simulink model "drawWorks_Sim_DriveBlk"  (R2017b)
settings: Solver=ode23t  StartTime=0.0  StopTime=30  FixedStep=Ts  MaxStep=1e-4  RelTol=1e-3  AbsTol=1e-3  EnableMultiTasking=on
PreLoadFcn:
  | addpath('./Images');
  | addpath('./Simscape_Pulley_Library');
InitFcn:
  | DrawworksParameters();
values from neighbouring files (symbols this model uses):
  n = 6    [DrawworksParameters.m]
  Ts = 1.5e-4    (= 0.00015)    [DrawworksParameters.m]
  Tssc = 10*Ts    (= 0.0015)    [DrawworksParameters.m]
undefined symbols (not defined in the file or in its folder): Drum, Tackle
libraries: fl_lib x19, CustomComponents_lib x11, nesl_utility x5, sdl_lib x3, powerlib x2, electricdrivelib x1
Description:
  | Copyright 2008-2016 The MathWorks, Inc.
settings Model: ExtModeAutoUpdateStatusClock=off  Creator=MathWorks  LastModifiedBy=jlesage
settings DataIOCC: LimitDataPoints=on  SaveFormat=Array  SignalLoggingSaveFormat=ModelDataLogs  SaveOutput=off  SignalLogging=off  SaveTime=off  SignalLoggingName=sigsOut
settings OptimizationCC: ExpressionDepthLimit=2147483647  InitFltsAndDblsToZero=on  LifeSpan=inf
settings DebuggingCC: UnderspecifiedInitializationDetection=Classic  MergeDetectMultiDrivingBlocksExec=none  CheckExecutionContextPreStartOutputMsg=on  CheckExecutionContextRuntimeOutputMsg=on  SignalResolutionControl=TryResolveAllWithWarning  MultiTaskDSMMsg=warning  MultiTaskCondExecSysMsg=none  FcnCallInpInsideContextMsg=warning  StateNameClashWarn=warning  SFUnexpectedBacktrackingDiag=warning  SFNoUnconditionalDefaultTransitionDiag=warning  SFExecutionAtInitializationDiag=none
settings HardwareCC: ProdBitPerPointer=32  ProdBitPerSizeT=32  ProdBitPerPtrDiffT=32  ProdLargestAtomicFloat=None  ProdIntDivRoundTo=Undefined  ProdEndianess=Unspecified  ProdWordSize=32  ProdHWDeviceType=32-bit Generic  TargetUnknown=on
settings ModelReferenceCC: PropagateSignalLabelsOutOfModel=off
settings CodeAppCC: StateflowObjectComments=on
settings GRTTargetCC: TargetLangStandard=C89/C90 (ANSI)  GeneratePreprocessorConditionals=Disable all  CombineOutputUpdateFcns=off  GRTInterface=on
settings ConfigComp: CovMetricSettings=dw  CovHtmlReporting=on  CovSaveCumulativeToWorkspaceVar=on  CovSaveSingleToWorkspaceVar=on  CovExternalEMLEnable=off  CovSFcnEnable=off
settings SimscapeCC: SimscapeNormalizeSystem=off

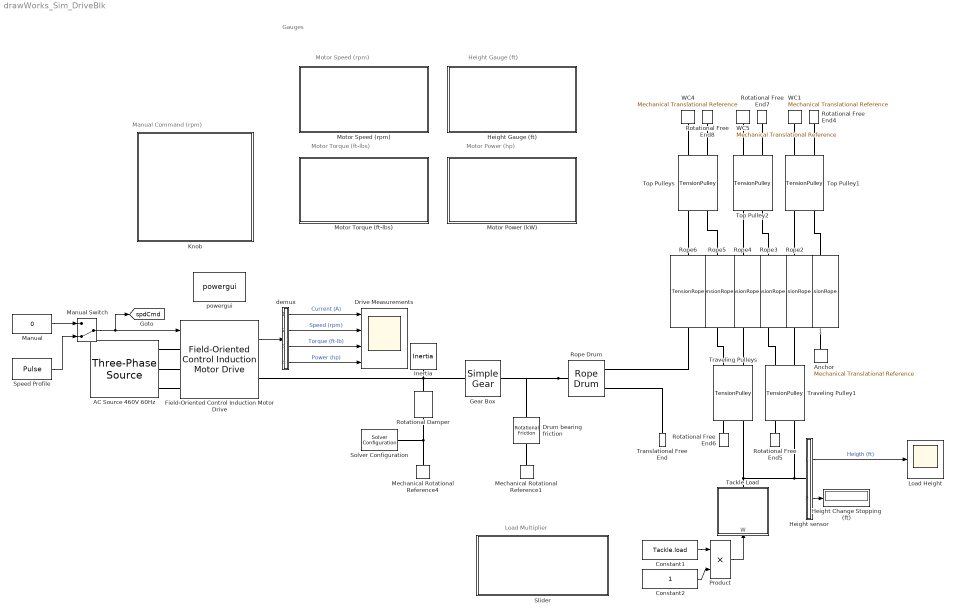
== system drawWorks_Sim_DriveBlk ==
  note: Gauges
  note: Motor Speed (rpm)
  note: Height Gauge (ft)
  note: Motor Torque (ft-lbs)
  note: Motor Power (hp)
  note: Manual Command (rpm)
  note: Load Multiplier
  1 : CustomComponents_lib/TensionRope  rope_stiff=Rope.stiffness N/m  damping=Rope.damping N/(m/s)  L0=10 m  mass=1 kg  s_specify=off  s_priority=High  s=0.08 m  s_nominal_specify=off  s_nominal_unit=m  s_nominal_value=1  L_specify=off  L_priority=High  L=1 m  L_nominal_specify=off  L_nominal_unit=m  L_nominal_value=1  f_specify=on  f_priority=High  f=Tackle.load/n N  f_nominal_specify=off  f_nominal_unit=N  f_nominal_value=1  v_specify=off  v_priority=High  v=0 m/s  v_nominal_specify=off  v_nominal_unit=m/s  v_nominal_value=1  fd_specify=off  fd_priority=High  fd=0 N  fd_nominal_specify=off  fd_nominal_unit=N  fd_nominal_value=1  fs_specify=off  fs_priority=High  fs=0 N  fs_nominal_specify=off  fs_nominal_unit=N  fs_nominal_value=1
  AC Source 460V 60Hz : powerlib/Electrical Sources/Three-Phase Source  InternalConnection=Yg  VoltagePhases=off  Voltage=2300  PhaseAngle=0  Voltage_phases=[25e3 25e3 25e3]/sqrt(3)  PhaseAngles_phases=[0 -120 +120]  Frequency=60  NonIdealSource=on  SpecifyImpedance=off  Resistance=0.02  Inductance=0.05e-3  ShortCircuitLevel=100e6  BaseVoltage=25e3  XRratio=7  BusType=swing  Pref=0  Qref=0  Prefabc=[10e3, 10e3, 10e3]  Qrefabc=[0, 0, 0]  Qmin=-inf  Qmax=inf
  Anchor : fl_lib/Mechanical/Translational Elements/Mechanical Translational Reference
  Constant1 : Constant  Value=Tackle.load
  Constant2 : Constant
  Drive Measurements : Scope  NumInputPorts=4
  Drum bearing friction : fl_lib/Mechanical/Rotational Elements/Rotational Friction  brkwy_trq=Drum.friction*1.1 N*m  brkwy_vel=0.060623 rad/s  Col_trq=Drum.friction N*m  visc_coef=Drum.viscous N*m/(rad/s)  w_specify=on  w_priority=Low  w=0 rad/s  w_nominal_specify=off  w_nominal_unit=rad/s  w_nominal_value=1  t_specify=off  t_priority=High  t=0 N*m  t_nominal_specify=off  t_nominal_unit=N*m  t_nominal_value=1
      settings: SourceProductName=Simscape
  Field-Oriented Control Induction Motor Drive : electricdrivelib/AC drives/Field-Oriented Control Induction Motor Drive  ReferenceFrame=Rotor  IterativeDiscreteModel=Forward Euler  Pn=2250*746  Vn=2300  fn=60  Rs=0.029  Lls=0.226/(2*pi*60)  Lms=13.04/(2*pi*60)  Rr=0.022  Llr=0.226/(2*pi*60)  ia=0  pha=0  ib=0  phb=0  ic=0  phc=0  J=3.1  Friction=0.08  p=2  slip=1  thdeg=0  Rsnb_rec=10e3  Csnb_rec=20e-9  Ron_rec=1e-3  Vf_rec=1.3  cap_bus=7500e-6  Rbrake=8  fbrake=4000  activationVoltage=700  shutdownVoltage=660  sourceFrequency=60  deviceType=IGBT / Diodes  Ron_inv=1e-3  Vf_inv=0.8  Vfd_inv=0.8  Tf=1e-6  Tt=2e-6  Tf_GTO=10e-6  Tt_GTO=20e-6  Rsnb_inv=5e3  Csnb_inv=inf  regulationType=Speed regulation  Acc=750  Dec=-750  kp_sc=300  ki_sc=2000  fc_sc=1000  Tsc=Ts  Tmin=-30000  Tmax=30000  in_flux=0.73  nf=0.73  kp_fc=50  ki_fc=30  freqc_fc=27  fluxmin=-2  fluxmax=2  modulationType=Hysteresis  h=10  kp_Id=5  ki_Id=100  kp_Iq=5  ki_Iq=100  fc_bus=50  car_freq=20000  freq_max=20000  Tvect=Ts  baseSampleTime=Ts  outputBusMode=Single output bus  busLabels=off  MechanicalLoad=Mechanical rotational port  modelDetailLevel=Average  driveType=AC3  AverageValue=on
      settings: SourceProductName=Simscape Power Systems  SourceProductBaseCode=PS
  Gear Box : sdl_lib/Gears/Simple Gear  ratio=10  rotation_direction=2  friction_model=1  T_noload=0.1 N*m  T_nom=5 N*m  efficiency_nom=0.8  efficiency=0.8  mu_visc=[ 0 0 ] N*m/(rad/s)  w_thr=0.01 rad/s  pwr_thr=0.001 W  temperature_TLU=[ 280 300 320 ] K  load_TLU=[ 1 5 10 ] N*m  efficiency_TLU=[ 0.95 0.9 0.85 ]  efficiency_TLU2=[ 0.85 0.8 0.75; 0.95 0.9 0.85; 0.85 0.8 0.7 ]  thermal_mass=50 J/K  T_init=300 K
      settings: SourceProductName=Simscape Driveline
  Height sensor : Subsystem
  Height Change Stopping (ft) : Display
  Height Gauge (ft) : Subsystem  DialogController=hmiCreateDDGDialog  IsWebBlock=on  mask(MathWorksWebBlock){webBlockId=c5aa380d-2f8e-459f-9f85-e92ca37c4779, webBlockType=semicirculargauge, ShowInLibBrowser=on, ShowInitialText=on, HMISrcModelName=drawWorks_Sim_DriveBlk}
      mask prompts: webBlockId "WebBlock Id"; webBlockType "WebBlock Type"; HMISrcModelName "Source Model"
      mask Help: helpview([docroot '/mapfiles/simulink.map'], 'hmi_half_gauge')
      mask Display:
      | if strcmp(get_param(bdroot(gcb),'BlockDiagramType'), 'library')
      |     image([(matlabroot) '/toolbox/simulink/hmi/icons/SemicircularGauge.png']);
      | end
  Inertia : fl_lib/Mechanical/Rotational Elements/Inertia  inertia=0.01 kg*m^2  w_specify=off  w_priority=High  w=0 rad/s  w_nominal_specify=off  w_nominal_unit=rad/s  w_nominal_value=1  t_specify=off  t_priority=High  t=0 N*m  t_nominal_specify=off  t_nominal_unit=N*m  t_nominal_value=1
  Knob : Subsystem  DialogController=hmiCreateDDGDialog  IsWebBlock=on  mask(MWDashboardBlock){webBlockId=b3dd6734-29cc-4e38-a886-5498566ea54e, webBlockType=continuousknob, ShowInLibBrowser=on, ShowInitialText=on, HMISrcModelName=drawWorks_Sim_DriveBlk}
      mask prompts: webBlockId "WebBlock Id"; webBlockType "WebBlock Type"; HMISrcModelName "Source Model"
      mask help: SimulinkHMI:dialogs:ContinuousKnobDialogDesc
      mask Help: helpview([docroot '/mapfiles/simulink.map'], 'hmi_knob')
      mask Display:
      | if strcmp(get_param(bdroot(gcb),'BlockDiagramType'), 'library')
      |     image([(matlabroot) '/toolbox/simulink/hmi/icons/ContinuousKnob.png']);
      | end
  Load Height : Scope
  Manual : Constant  Value=0
  Manual Switch : ManualSwitch  CurrentSetting=0
  Mechanical Rotational Reference1 : fl_lib/Mechanical/Rotational Elements/Mechanical Rotational Reference
  Mechanical Rotational Reference4 : fl_lib/Mechanical/Rotational Elements/Mechanical Rotational Reference
  Motor Power (kW) : Subsystem  DialogController=hmiCreateDDGDialog  IsWebBlock=on  mask(MathWorksWebBlock){webBlockId=19b5fd22-3d9e-453c-98f3-af57f09a4a2a, webBlockType=semicirculargauge, ShowInLibBrowser=on, ShowInitialText=on, HMISrcModelName=drawWorks_Sim_DriveBlk}
      mask prompts: webBlockId "WebBlock Id"; webBlockType "WebBlock Type"; HMISrcModelName "Source Model"
      mask Help: helpview([docroot '/mapfiles/simulink.map'], 'hmi_half_gauge')
      mask Display:
      | if strcmp(get_param(bdroot(gcb),'BlockDiagramType'), 'library')
      |     image([(matlabroot) '/toolbox/simulink/hmi/icons/SemicircularGauge.png']);
      | end
  Motor Speed (rpm) : Subsystem  DialogController=hmiCreateDDGDialog  IsWebBlock=on  mask(MathWorksWebBlock){webBlockId=7eba74a7-8cbb-4d45-95db-04e3d24d85db, webBlockType=semicirculargauge, ShowInLibBrowser=on, ShowInitialText=on, HMISrcModelName=drawWorks_Sim_DriveBlk}
      mask prompts: webBlockId "WebBlock Id"; webBlockType "WebBlock Type"; HMISrcModelName "Source Model"
      mask Help: helpview([docroot '/mapfiles/simulink.map'], 'hmi_half_gauge')
      mask Display:
      | if strcmp(get_param(bdroot(gcb),'BlockDiagramType'), 'library')
      |     image([(matlabroot) '/toolbox/simulink/hmi/icons/SemicircularGauge.png']);
      | end
  Motor Torque (ft-lbs) : Subsystem  DialogController=hmiCreateDDGDialog  IsWebBlock=on  mask(MathWorksWebBlock){webBlockId=3687f525-ad22-450b-a80e-b9211f80e0d5, webBlockType=semicirculargauge, ShowInLibBrowser=on, ShowInitialText=on, HMISrcModelName=drawWorks_Sim_DriveBlk}
      mask prompts: webBlockId "WebBlock Id"; webBlockType "WebBlock Type"; HMISrcModelName "Source Model"
      mask Help: helpview([docroot '/mapfiles/simulink.map'], 'hmi_half_gauge')
      mask Display:
      | if strcmp(get_param(bdroot(gcb),'BlockDiagramType'), 'library')
      |     image([(matlabroot) '/toolbox/simulink/hmi/icons/SemicircularGauge.png']);
      | end
  Product : Product
  Rope Drum : sdl_lib/Couplings & Drives/Rope Drum  r_drum=Drum.radius m  windup=2  check_tension=1  b_drum=0 N*m/(rad/s)  model_inertia=1  inertia=Drum.inertia kg*m^2  initial_velocity=0 rad/s
      settings: SourceProductName=Simscape Driveline  SourceProductBaseCode=LD
  Rope{2..6} (5 alike) : CustomComponents_lib/TensionRope  rope_stiff=Rope.stiffness N/m  damping=Rope.damping N/(m/s)  L0=10 m  mass=1 kg  s_specify=off  s_priority=High  s=0.08 m  s_nominal_specify=off  s_nominal_unit=m  s_nominal_value=1  L_specify=off  L_priority=High  L=1 m  L_nominal_specify=off  L_nominal_unit=m  L_nominal_value=1  f_specify=on  f_priority=High  f=Tackle.load/n N  f_nominal_specify=off  f_nominal_unit=N  f_nominal_value=1  v_specify=off  v_priority=High  v=0 m/s  v_nominal_specify=off  v_nominal_unit=m/s  v_nominal_value=1  fd_specify=off  fd_priority=High  fd=0 N  fd_nominal_specify=off  fd_nominal_unit=N  fd_nominal_value=1  fs_specify=off  fs_priority=High  fs=0 N  fs_nominal_specify=off  fs_nominal_unit=N  fs_nominal_value=1
  Rotational Damper : fl_lib/Mechanical/Rotational Elements/Rotational Damper  D=0.001 N*m/(rad/s)  w_specify=off  w_priority=High  w=0 rad/s  w_nominal_specify=off  w_nominal_unit=rad/s  w_nominal_value=1  t_specify=off  t_priority=High  t=0 N*m  t_nominal_specify=off  t_nominal_unit=N*m  t_nominal_value=1
  Rotational Free End{4..8} (5 alike) : fl_lib/Mechanical/Rotational Elements/Rotational Free End  w_specify=off  w_priority=High  w=0 rad/s  w_nominal_specify=off  w_nominal_unit=rad/s  w_nominal_value=1
      settings: SourceProductName=Simscape  SourceProductBaseCode=SS
  Slider : Subsystem  DialogController=hmiCreateDDGDialog  IsWebBlock=on  mask(MWDashboardBlock){webBlockId=0993a495-73f7-4df6-a704-f2e0e4754f77, webBlockType=slider, ShowInLibBrowser=on, ShowInitialText=on, HMISrcModelName=drawWorks_Sim_DriveBlk}
      mask prompts: webBlockId "WebBlock Id"; webBlockType "WebBlock Type"; HMISrcModelName "Source Model"
      mask help: SimulinkHMI:dialogs:SliderDialogDesc
      mask Help: helpview([docroot '/mapfiles/simulink.map'], 'hmi_slider')
      mask Display:
      | if strcmp(get_param(bdroot(gcb),'BlockDiagramType'), 'library')
      |     image([(matlabroot) '/toolbox/simulink/hmi/icons/Slider.png']);
      | end
  Solver Configuration : nesl_utility/Solver Configuration  PhysicalDomain=network_engine_domain  SubClassName=solver  LeftPortType=input  RightPortType=generic  Accelerate=off  Tones=[]  Harmonics=[]  SimulateNoise=off  Profile=off  UseLocalSampling=off  EnableSwitchedLinearOptims=on  FrequencyDomain=off  UseCCode=off  RelTol=0.001  AbsTol=1e-06  MinStep=1e-09  ToWorkspace=off  RevertToSquareIcSolve=off  NumHomotopyIterations=100  PhasorMode=off  PhasorModeNumHarmonics=1  DoDC=off  ResidualTolerance=1e-09  UseLocalSolver=on  LocalSolverChoice=NE_BACKWARD_EULER_ADVANCER  LocalSolverSampleTime=Tssc  DoFixedCost=on  MaxNonlinIter=3  MaxModeIter=2  LinearAlgebra=Sparse  DelaysMemoryBudget=1024  AutomaticFiltering=on  FilteringTimeConstant=0.001
  Speed Profile : DiscretePulseGenerator  PulseType=Time based  Amplitude=1250  Period=15  PulseWidth=60  PhaseDelay=2.5
  Tackle Load : Subsystem
      mask Display: image('tackle.jpg')
  Top Pulley1 : CustomComponents_lib/TensionPulley  radius=Pulley.radius m  b_damp=Pulley.viscous N*m/(rad/s)  inertia=Pulley.inertia kg*m^2  mass=1 kg  mu_s=1  f_A_specify=off  f_A_priority=High  f_A=0 N  f_A_nominal_specify=off  f_A_nominal_unit=N  f_A_nominal_value=1  f_B_specify=off  f_B_priority=High  f_B=0 N  f_B_nominal_specify=off  f_B_nominal_unit=N  f_B_nominal_value=1  f_C_specify=off  f_C_priority=High  f_C=0 N  f_C_nominal_specify=off  f_C_nominal_unit=N  f_C_nominal_value=1  tau_specify=off  tau_priority=High  tau=0 N*m  tau_nominal_specify=off  tau_nominal_unit=N*m  tau_nominal_value=1  w_specify=off  w_priority=High  w=0 rad/s  w_nominal_specify=off  w_nominal_unit=rad/s  w_nominal_value=1  v_specify=off  v_priority=High  v=0 m/s  v_nominal_specify=off  v_nominal_unit=m/s  v_nominal_value=1
  Top Pulley2 : CustomComponents_lib/TensionPulley  radius=Pulley.radius m  b_damp=Pulley.viscous N*m/(rad/s)  inertia=Pulley.inertia kg*m^2  mass=1 kg  mu_s=1  f_A_specify=off  f_A_priority=High  f_A=0 N  f_A_nominal_specify=off  f_A_nominal_unit=N  f_A_nominal_value=1  f_B_specify=off  f_B_priority=High  f_B=0 N  f_B_nominal_specify=off  f_B_nominal_unit=N  f_B_nominal_value=1  f_C_specify=off  f_C_priority=High  f_C=0 N  f_C_nominal_specify=off  f_C_nominal_unit=N  f_C_nominal_value=1  tau_specify=off  tau_priority=High  tau=0 N*m  tau_nominal_specify=off  tau_nominal_unit=N*m  tau_nominal_value=1  w_specify=off  w_priority=High  w=0 rad/s  w_nominal_specify=off  w_nominal_unit=rad/s  w_nominal_value=1  v_specify=off  v_priority=High  v=0 m/s  v_nominal_specify=off  v_nominal_unit=m/s  v_nominal_value=1
  Top Pulleys : CustomComponents_lib/TensionPulley  radius=Pulley.radius m  b_damp=Pulley.viscous N*m/(rad/s)  inertia=Pulley.inertia kg*m^2  mass=1 kg  mu_s=1  f_A_specify=off  f_A_priority=High  f_A=0 N  f_A_nominal_specify=off  f_A_nominal_unit=N  f_A_nominal_value=1  f_B_specify=off  f_B_priority=High  f_B=0 N  f_B_nominal_specify=off  f_B_nominal_unit=N  f_B_nominal_value=1  f_C_specify=off  f_C_priority=High  f_C=0 N  f_C_nominal_specify=off  f_C_nominal_unit=N  f_C_nominal_value=1  tau_specify=off  tau_priority=High  tau=0 N*m  tau_nominal_specify=off  tau_nominal_unit=N*m  tau_nominal_value=1  w_specify=off  w_priority=High  w=0 rad/s  w_nominal_specify=off  w_nominal_unit=rad/s  w_nominal_value=1  v_specify=off  v_priority=High  v=0 m/s  v_nominal_specify=off  v_nominal_unit=m/s  v_nominal_value=1
  Translational Free End : fl_lib/Mechanical/Translational Elements/Translational Free End  v_specify=off  v_priority=High  v=0 m/s  v_nominal_specify=off  v_nominal_unit=m/s  v_nominal_value=1
      settings: SourceProductName=Simscape  SourceProductBaseCode=SS
  Traveling Pulley1 : CustomComponents_lib/TensionPulley  radius=Pulley.radius m  b_damp=Pulley.viscous N*m/(rad/s)  inertia=Pulley.inertia kg*m^2  mass=1 kg  mu_s=1  f_A_specify=off  f_A_priority=High  f_A=0 N  f_A_nominal_specify=off  f_A_nominal_unit=N  f_A_nominal_value=1  f_B_specify=off  f_B_priority=High  f_B=0 N  f_B_nominal_specify=off  f_B_nominal_unit=N  f_B_nominal_value=1  f_C_specify=off  f_C_priority=High  f_C=0 N  f_C_nominal_specify=off  f_C_nominal_unit=N  f_C_nominal_value=1  tau_specify=off  tau_priority=High  tau=0 N*m  tau_nominal_specify=off  tau_nominal_unit=N*m  tau_nominal_value=1  w_specify=off  w_priority=High  w=0 rad/s  w_nominal_specify=off  w_nominal_unit=rad/s  w_nominal_value=1  v_specify=off  v_priority=High  v=0 m/s  v_nominal_specify=off  v_nominal_unit=m/s  v_nominal_value=1
  Traveling Pulleys : CustomComponents_lib/TensionPulley  radius=Pulley.radius m  b_damp=Pulley.viscous N*m/(rad/s)  inertia=Pulley.inertia kg*m^2  mass=1 kg  mu_s=1  f_A_specify=off  f_A_priority=High  f_A=0 N  f_A_nominal_specify=off  f_A_nominal_unit=N  f_A_nominal_value=1  f_B_specify=off  f_B_priority=High  f_B=0 N  f_B_nominal_specify=off  f_B_nominal_unit=N  f_B_nominal_value=1  f_C_specify=off  f_C_priority=High  f_C=0 N  f_C_nominal_specify=off  f_C_nominal_unit=N  f_C_nominal_value=1  tau_specify=off  tau_priority=High  tau=0 N*m  tau_nominal_specify=off  tau_nominal_unit=N*m  tau_nominal_value=1  w_specify=off  w_priority=High  w=0 rad/s  w_nominal_specify=off  w_nominal_unit=rad/s  w_nominal_value=1  v_specify=off  v_priority=High  v=0 m/s  v_nominal_specify=off  v_nominal_unit=m/s  v_nominal_value=1
  WC1 : fl_lib/Mechanical/Translational Elements/Mechanical Translational Reference
  WC4 : fl_lib/Mechanical/Translational Elements/Mechanical Translational Reference
  WC5 : fl_lib/Mechanical/Translational Elements/Mechanical Translational Reference
  demux : Subsystem
  powergui : powerlib/powergui  Priority=2  SimulationMode=Discrete  SampleTime=Ts  frequency=60  Iterations=50  frequencyindice=60  Pbase=100e6  ErrMax=1e-4  UnitsV=kV  UnitsW=MW  buscounter=0  FunctionMessages=off  echomessages=off  EnableUseOfTLC=off  CurrentSourceSwitches=off  DisableSnubberDevices=off  DisableRonSwitches=off  DisableVfSwitches=off  DisplayEquations=off  SolverType=Tustin/Backward Euler (TBE)  Interpol=off  ExternalGateDelay=off  methode=off  Ts=100  x0status=blocks  SPID=on  SwTol=0  HookPort=off  RestoreLinks=warning  ResistiveCurrentMeasurement=off  Frange=[0:2:500]  Ylog=off  Xlog=on  ShowGrid=off  save=off  variable=ZData  structure=simout  ZoomFFT=on  StartTime=0.05  cycles=7  DisplayStyle=1  fundamental=60  FreqAxis=off  MaxFrequency=20000  frequencyindicesteady=1  RmsSteady=1  display=off
  tag scope: spdCmd=global
  wires:
  demux/1(i_a) -> Drive Measurements/1  "Current (A)"
  demux/2(speed) -> Drive Measurements/2  "Speed (rpm)"
  demux/3(Tem) -> Drive Measurements/3  "Torque (ft-lb)"
  Field-Oriented Control Induction Motor Drive/1 -> demux/1(motor)
  Height sensor/1(x) -> Load Height/1  "Heigth (ft)"
  Manual/1 -> Manual Switch/1
  Manual Switch/1 -> Field-Oriented Control Induction Motor Drive/1, [spdCmd]
  Speed Profile/1 -> Manual Switch/2
  demux/4(P) -> Drive Measurements/4  "Power (hp)"
  Height sensor/2(h) -> Height Change Stopping (ft)/1
  Constant1/1 -> Product/1
  Product/1 -> Tackle Load/1(W)
  Constant2/1 -> Product/2
  connections:
  Tackle Load/RConn1 -- Traveling Pulleys/LConn1 -- Traveling Pulley1/LConn1 -- Height sensor/LConn1
  Rope Drum/LConn1 -- Drum bearing friction/LConn1 -- Gear Box/RConn1
  Inertia/LConn1 -- Field-Oriented Control Induction Motor Drive/RConn1 -- Rotational Damper/LConn1 -- Gear Box/LConn1
  Rope5/RConn1 -- Top Pulleys/RConn2
  WC1/LConn1 -- Top Pulley1/LConn1
  Rope6/RConn1 -- Top Pulleys/RConn1
  Anchor/LConn1 -- 1/LConn1
  Top Pulley2/RConn2 -- Rope3/RConn1
  Rope5/LConn1 -- Traveling Pulleys/RConn2
  WC5/LConn1 -- Top Pulley2/LConn1
  Rope Drum/RConn1 -- Translational Free End/LConn1
  Rotational Free End6/LConn1 -- Traveling Pulleys/LConn2
  Rope4/LConn1 -- Traveling Pulleys/RConn1
  Rope Drum/RConn2 -- Rope6/LConn1
  Rotational Free End4/LConn1 -- Top Pulley1/LConn2
  Rotational Damper/RConn1 -- Mechanical Rotational Reference4/LConn1 -- Solver Configuration/RConn1
  Rope4/RConn1 -- Top Pulley2/RConn1
  Rope2/RConn1 -- Top Pulley1/RConn1
  WC4/LConn1 -- Top Pulleys/LConn1
  Drum bearing friction/RConn1 -- Mechanical Rotational Reference1/LConn1
  1/RConn1 -- Top Pulley1/RConn2
  Rotational Free End5/LConn1 -- Traveling Pulley1/LConn2
  Rotational Free End7/LConn1 -- Top Pulley2/LConn2
  Rope3/LConn1 -- Traveling Pulley1/RConn2
  Rotational Free End8/LConn1 -- Top Pulleys/LConn2
  Rope2/LConn1 -- Traveling Pulley1/RConn1
  AC Source 460V 60Hz/RConn1 -- Field-Oriented Control Induction Motor Drive/LConn1
  AC Source 460V 60Hz/RConn3 -- Field-Oriented Control Induction Motor Drive/LConn3
  AC Source 460V 60Hz/RConn2 -- Field-Oriented Control Induction Motor Drive/LConn2

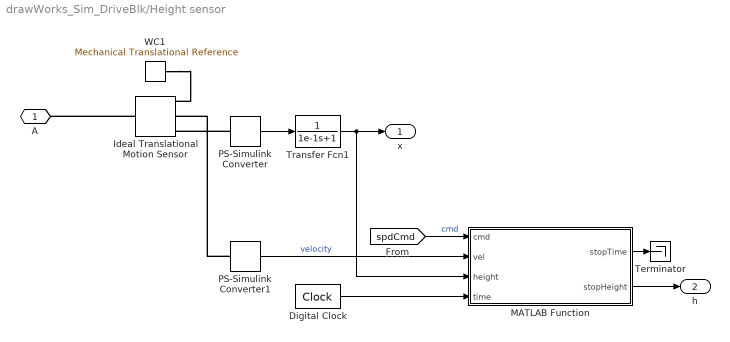
== system drawWorks_Sim_DriveBlk/Height sensor ==
  Digital Clock : DigitalClock  SampleTime=Tssc
  Ideal Translational Motion Sensor : fl_lib/Mechanical/Mechanical Sensors/Ideal Translational Motion Sensor  offset=0 m
  MATLAB Function : MATLAB Function  TreatAsAtomicUnit=on  SystemSampleTime=Tssc
  PS-Simulink Converter : nesl_utility/PS-Simulink Converter  PhysicalDomain=network_engine_domain  SubClassName=ps_output  LeftPortType=input  RightPortType=output  PseudoPeriodic=off  Frequencies=[]  Unit=ft  AffineConversion=off
  PS-Simulink Converter1 : nesl_utility/PS-Simulink Converter  PhysicalDomain=network_engine_domain  SubClassName=ps_output  LeftPortType=input  RightPortType=output  PseudoPeriodic=off  Frequencies=[]  Unit=ft/s  AffineConversion=off
  Terminator : Terminator
  Transfer Fcn1 : TransferFcn  Denominator=[1e-1 1]
  WC1 : fl_lib/Mechanical/Translational Elements/Mechanical Translational Reference
  A : PMIOPort  Port=1  Side=Left
  x : Outport
  h : Outport  Port=2
  wires:
  PS-Simulink Converter/1 -> Transfer Fcn1/1
  Transfer Fcn1/1 -> MATLAB Function/3(height), x/1
  PS-Simulink Converter1/1 -> MATLAB Function/2(vel)  "velocity"
  [spdCmd] -> MATLAB Function/1(cmd)  "cmd"
  Digital Clock/1 -> MATLAB Function/4(time)
  MATLAB Function/2(stopHeight) -> h/1
  MATLAB Function/1(stopTime) -> Terminator/1
  connections:
  PS-Simulink Converter/LConn1 -- Ideal Translational Motion Sensor/RConn3
  Ideal Translational Motion Sensor/LConn1 -- A/RConn1
  WC1/LConn1 -- Ideal Translational Motion Sensor/RConn1
  PS-Simulink Converter1/LConn1 -- Ideal Translational Motion Sensor/RConn2

== system drawWorks_Sim_DriveBlk/Height Gauge (ft) ==

== system drawWorks_Sim_DriveBlk/Knob ==

== system drawWorks_Sim_DriveBlk/Motor Power (kW) ==

== system drawWorks_Sim_DriveBlk/Motor Speed (rpm) ==

== system drawWorks_Sim_DriveBlk/Motor Torque (ft-lbs) ==

== system drawWorks_Sim_DriveBlk/Slider ==

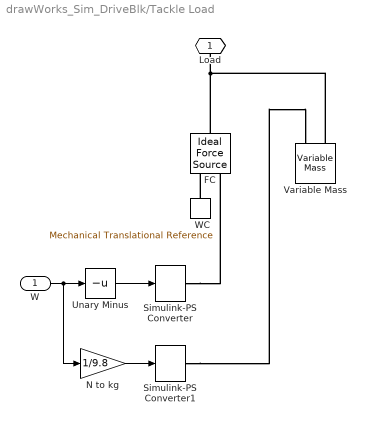
== system drawWorks_Sim_DriveBlk/Tackle Load ==
  W : Inport
  FC : fl_lib/Mechanical/Mechanical Sources/Ideal Force Source
  N to kg : Gain  Gain=1/9.8
  Simulink-PS Converter : nesl_utility/Simulink-PS Converter  PhysicalDomain=network_engine_domain  SubClassName=ps_input  LeftPortType=input  RightPortType=output  PseudoPeriodic=off  Frequencies=[]  NoiseDistribution=none  NoiseParameters=[]  Unit=N  AffineConversion=off  FilteringAndDerivatives=zero  SimscapeFilterOrder=2  InputFilterTimeConstant=0.001  UdotUserProvided=1
  Simulink-PS Converter1 : nesl_utility/Simulink-PS Converter  PhysicalDomain=network_engine_domain  SubClassName=ps_input  LeftPortType=input  RightPortType=output  PseudoPeriodic=off  Frequencies=[]  NoiseDistribution=none  NoiseParameters=[]  Unit=kg  AffineConversion=off  FilteringAndDerivatives=zero  SimscapeFilterOrder=2  InputFilterTimeConstant=0.001  UdotUserProvided=1
  Unary Minus : UnaryMinus
  Variable Mass : sdl_lib/Inertias & Loads/Variable Mass  minimum_mass=0.1 kg  p_specify=on  p_priority=High  p=0 m*kg/s  p_nominal_specify=off  p_nominal_unit=m*kg/s  p_nominal_value=1
      settings: SourceProductName=Simscape Driveline  SourceProductBaseCode=LD
  WC : fl_lib/Mechanical/Translational Elements/Mechanical Translational Reference
  Load : PMIOPort  Port=1  Side=Right
  wires:
  W/1 -> Unary Minus/1, N to kg/1
  Unary Minus/1 -> Simulink-PS Converter/1
  N to kg/1 -> Simulink-PS Converter1/1
  connections:
  WC/LConn1 -- FC/RConn2
  Simulink-PS Converter/RConn1 -- FC/RConn1
  FC/LConn1 -- Variable Mass/LConn2 -- Load/RConn1
  Simulink-PS Converter1/RConn1 -- Variable Mass/LConn1

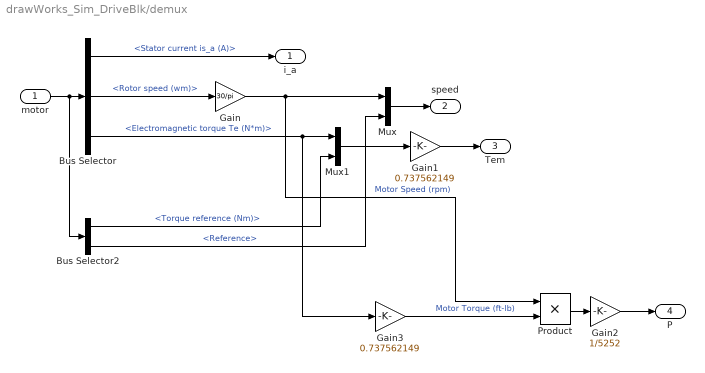
== system drawWorks_Sim_DriveBlk/demux ==
  motor : Inport
  Bus Selector : BusSelector  OutputSignals=Motor.Stator measurements.Stator current is_a (A),Motor.Mechanical.Rotor speed (wm),Motor.Mechanical.Electromagnetic torque Te (N*m)
  Bus Selector2 : BusSelector  OutputSignals=Ctrl.Torque reference (Nm),Ctrl.Reference
  Gain : Gain  Gain=30/pi  SaturateOnIntegerOverflow=on  OutDataTypeStr=Inherit: Same as input  ParamDataTypeStr=Inherit: Same as input
  Gain1 : Gain  Gain=0.737562149  SaturateOnIntegerOverflow=on  OutDataTypeStr=Inherit: Same as input  ParamDataTypeStr=Inherit: Same as input
  Gain2 : Gain  Gain=1/5252  SaturateOnIntegerOverflow=on  OutDataTypeStr=Inherit: Same as input  ParamDataTypeStr=Inherit: Same as input
  Gain3 : Gain  Gain=0.737562149  SaturateOnIntegerOverflow=on  OutDataTypeStr=Inherit: Same as input  ParamDataTypeStr=Inherit: Same as input
  Mux : Mux  Inputs=2
  Mux1 : Mux  Inputs=2
  Product : Product
  i_a : Outport
  speed : Outport  Port=2
  Tem : Outport  Port=3
  P : Outport  Port=4
  wires:
  motor/1 -> Bus Selector2/1, Bus Selector/1
  Mux/1 -> speed/1
  Mux1/1 -> Gain1/1
  Bus Selector/3 -> Gain3/1, Mux1/1  "<Electromagnetic torque Te (N*m)>"
  Bus Selector/2 -> Gain/1  "<Rotor speed (wm)>"
  Bus Selector/1 -> i_a/1  "<Stator current is_a (A)>"
  Gain/1 -> Product/1, Mux/1  "Motor Speed (rpm)"
  Bus Selector2/2 -> Mux/2  "<Reference>"
  Bus Selector2/1 -> Mux1/2  "<Torque reference (Nm)>"
  Gain1/1 -> Tem/1
  Gain2/1 -> P/1
  Product/1 -> Gain2/1
  Gain3/1 -> Product/2  "Motor Torque (ft-lb)"

== matlab function drawWorks_Sim_DriveBlk/Height sensor/MATLAB Function ==
  data: cmd input; stopTime output; vel input; height input; time input; stopHeight output
function [stopTime,stopHeight] = fcn(cmd,vel,height,time)

persistent timeElapse
persistent measTime
persistent timeStart
persistent prevCmd
persistent heightElapse
persistent heightStart

if isempty(timeElapse) || time < 1
    timeElapse = 0;
    measTime = 0;
    timeStart = time;
    prevCmd = 0;
    heightElapse = 0;
    heightStart = 0;
else  
    if cmd == 0 && abs(cmd-prevCmd) > 1e-1 && measTime == 0
        timeStart = time;
        heightStart = height;
        measTime = 1;
    end
    
    if measTime == 1 && abs(vel) < 1e-1
        timeElapse = time - timeStart;
        heightElapse = height - heightStart;
        measTime = 0;
    end
    
    % Update each step;
    prevCmd = cmd;
    
end

stopTime = timeElapse;
stopHeight = heightElapse;
